simulink model "discrete_test"  (R2022b)
settings: Solver=FixedStepAuto  StartTime=0.0  StopTime=10.0  FixedStep=0.0001  RelTol=1e-3
values from neighbouring files (symbols this model uses):
  a21 = 1/(2*m)*x30^2*FemP1/FemP2^2*exp(-x10/FemP2)    [ex5.m]
  a23 = -1/(m)*x30*FemP1/FemP2*exp(-x10/FemP2)    [ex5.m]
  a31 = 1/f1*exp(x10/f2)*(ki*u10+ci-x30)    [ex5.m]
  a33 = -f2/f1*exp(x10/f2)    [ex5.m]
  b31 = ki*f2/f1*exp(x10/f2)    [ex5.m]
  g = 9.81    [ex5.m]
  Kx = -acker(A, B(:,1), -sKx)    [ex5.m]
  Lo = acker(A', C', -sLo)    [ex5.m]
  u0 = -(a31*x1+a33*x3)/b31    [ex5.m]
  x1 = .003    (= 0.003)    [ex5.m]
  x2 = 0    [ex5.m]
  x3 = -(a21*x1+g)/a23    [ex5.m]
  xd = d-bd    (= 0.0192)    [ex5.m]
settings Model: Creator=MPatr  LastModifiedBy=MPatr

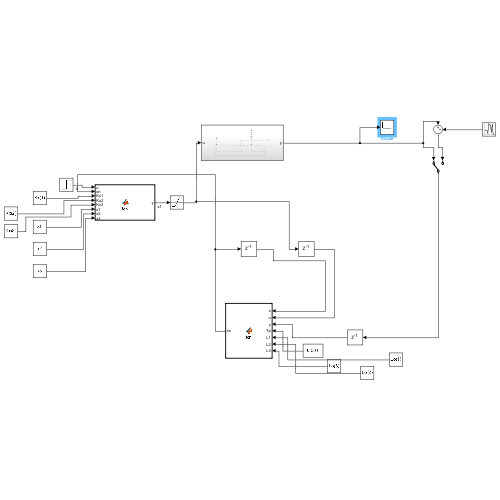
[thumbnail: Simulink's stored preview of the top-level diagram]
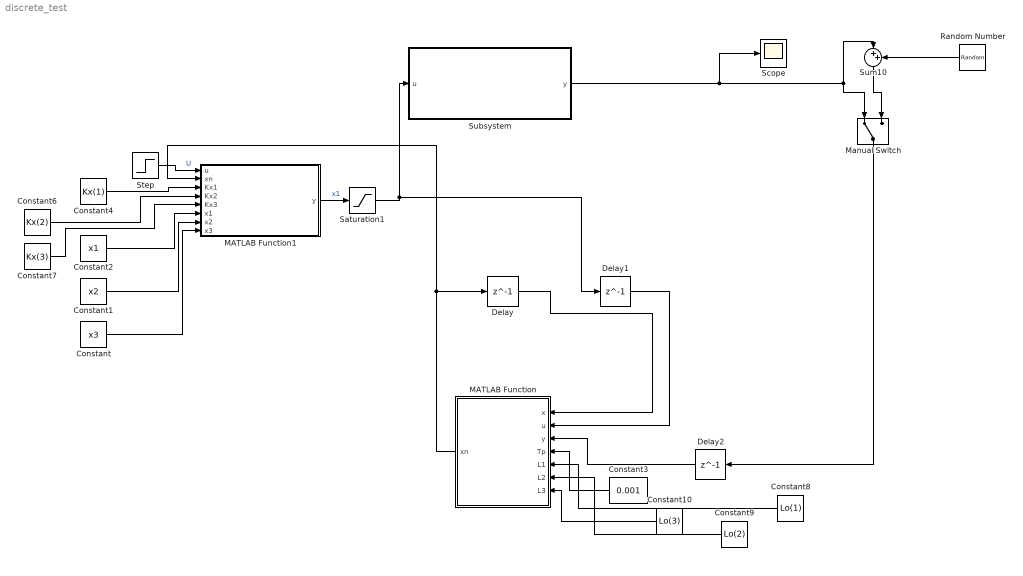
== system discrete_test ==
  Constant : Constant  Value=x3
  Constant1 : Constant  Value=x2
  Constant10 : Constant  Value=Lo(3)
  Constant2 : Constant  Value=x1
  Constant3 : Constant  Value=0.001
  Constant4 : Constant  Value=Kx(1)
  Constant6 : Constant  Value=Kx(2)
  Constant7 : Constant  Value=Kx(3)
  Constant8 : Constant  Value=Lo(1)
  Constant9 : Constant  Value=Lo(2)
  Delay : Delay  DelayLength=1
  Delay1 : Delay  DelayLength=1
  Delay2 : Delay  DelayLength=1
  MATLAB Function : MATLAB Function  TreatAsAtomicUnit=on
  MATLAB Function1 : MATLAB Function  TreatAsAtomicUnit=on
  Manual Switch : ManualSwitch
  Random Number : RandomNumber  Variance=.0000001
  Saturation1 : Saturate  UpperLimit=1  LowerLimit=0
  Scope : Scope
  Step : Step  Time=0  After=u0  SampleTime=0
  Subsystem : Subsystem
  Sum10 : Sum  Inputs=|++
  wires:
  Delay1/1 -> MATLAB Function/2(u)
  Delay2/1 -> MATLAB Function/3(y)
  MATLAB Function/1(xn) -> MATLAB Function1/2(xn), Delay/1
  Random Number/1 -> Sum10/2
  Manual Switch/1 -> Delay2/1
  Sum10/1 -> Manual Switch/2
  Delay/1 -> MATLAB Function/1(x)
  Constant3/1 -> MATLAB Function/4(Tp)
  MATLAB Function1/1(y) -> Saturation1/1  "x1"
  Step/1 -> MATLAB Function1/1(u)  "U"
  Constant2/1 -> MATLAB Function1/6(x1)
  Constant1/1 -> MATLAB Function1/7(x2)
  Constant/1 -> MATLAB Function1/8(x3)
  Constant4/1 -> MATLAB Function1/3(Kx1)
  Constant6/1 -> MATLAB Function1/4(Kx2)
  Constant7/1 -> MATLAB Function1/5(Kx3)
  Constant8/1 -> MATLAB Function/5(L1)
  Constant9/1 -> MATLAB Function/6(L2)
  Constant10/1 -> MATLAB Function/7(L3)
  Subsystem/1(y) -> Scope/1, Sum10/1, Manual Switch/1
  Saturation1/1 -> Subsystem/1(u), Delay1/1

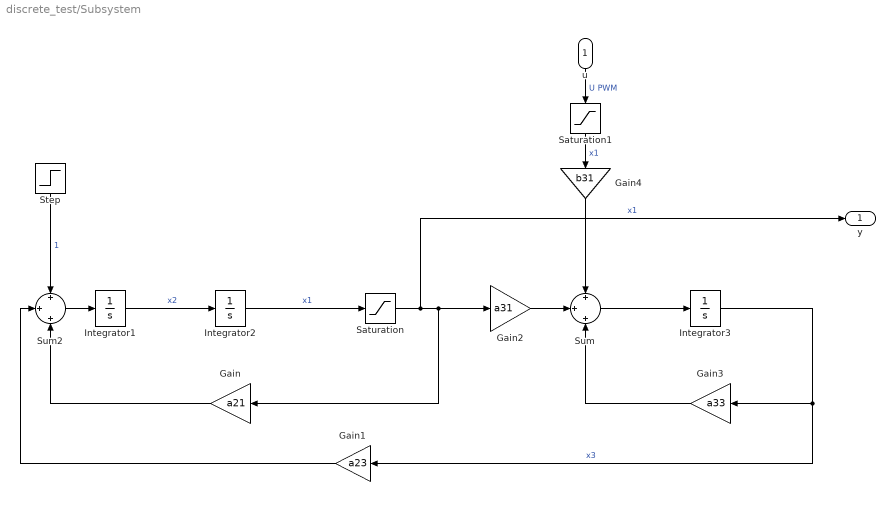
== system discrete_test/Subsystem ==
  u : Inport
  Gain : Gain  Gain=a21
  Gain1 : Gain  Gain=a23
  Gain2 : Gain  Gain=a31
  Gain3 : Gain  Gain=a33
  Gain4 : Gain  Gain=b31
  Integrator1 : Integrator
  Integrator2 : Integrator  InitialCondition=xd
  Integrator3 : Integrator
  Saturation : Saturate  UpperLimit=xd  LowerLimit=0
  Saturation1 : Saturate  UpperLimit=1  LowerLimit=0
  Step : Step  Time=0  After=g  SampleTime=0
  Sum : Sum  Inputs=+|+|+
  Sum2 : Sum  Inputs=+|+|+
  y : Outport
  wires:
  Step/1 -> Sum2/1  "1"
  Integrator1/1 -> Integrator2/1  "x2"
  Gain1/1 -> Sum2/2
  u/1 -> Saturation1/1  "U PWM"
  Saturation/1 -> y/1, Gain2/1, Gain/1  "x1"
  Integrator3/1 -> Gain3/1, Gain1/1  "x3"
  Gain/1 -> Sum2/3
  Gain2/1 -> Sum/2
  Gain3/1 -> Sum/3
  Sum2/1 -> Integrator1/1
  Sum/1 -> Integrator3/1
  Integrator2/1 -> Saturation/1  "x1"
  Gain4/1 -> Sum/1
  Saturation1/1 -> Gain4/1  "x1"

== matlab function discrete_test/MATLAB Function1 ==
  data: u input; y output; xn input; Kx1 input; Kx2 input; Kx3 input; x1 input; x2 input; x3 input
function y = fcn(u, xn, Kx1, Kx2, Kx3, x1, x2, x3)

y = u + [Kx1, Kx2, Kx3]*(xn-[x1; x2; x3]);

== matlab function discrete_test/MATLAB Function ==
  data: x input; u input; y input; Tp input; xn output; L1 input; L2 input; L3 input
function xn   = fcn(x, u, y, Tp, L1, L2, L3)

m = .00575;
g = 9.81;
FemP1 = .017521;
FemP2 = .0058231;
f1 = .00014142;
f2 = .0045626;
ki = 2.5165;
ci = .0243 * sign(4-2);
d = .0792;
bd = .06;
xd = d-bd;
x10 = .008;
x20 = 0;
x30 = .75;
u10 = 1/ki*(x30-ci);
% 0.2883767137

a21 = 1/(2*m)*x30^2*FemP1/FemP2^2*exp(-x10/FemP2); 
a23 = -1/(m)*x30*FemP1/FemP2*exp(-x10/FemP2); 
a31 = 1/f1*exp(x10/f2)*(ki*u10+ci-x30); 
a33 = -f2/f1*exp(x10/f2);
b31 = ki*f2/f1*exp(x10/f2);
A = [0 1 0; a21 0 a23; a31 0 a33];
B = [0 0; 0 g; b31 0];
C = [1 0 0];
D = 0;


% sLo = 200*ones(1,3)
Lo = [L1; L2; L3];

xn = (eye(3)+A*Tp)*x + B(:, 1)*Tp*u + Lo*Tp*(y-C*x);
